simulink model "ForceMeasurement"  (R2018a)
settings: Solver=ode4  StartTime=0.0  StopTime=inf  FixedStep=0.002  RelTol=1e-3  EnableMultiTasking=on
PostLoadFcn:
  | qc_set_target_type(getConfigSet(bdroot, 'QUARC Default Target Configuration'));
undefined symbols (not defined in the file or in its folder): HIL
libraries: quarc_library x9
Description:
  | This example is a simple analog loopback test. It sends a signal to analog output
  | channel #0 and then reads analog input channel #0. Wire analog output #0 to analog
  | input #0 to see the signal on the Scope. Change the amplitude of the signal and see
  | the change occur on the Scope.
settings Model: SimulationMode=external  ExtModeTrigDuration=10000  Creator=drmadill  LastModifiedBy=dogro
settings SolverCC: PositivePriorityOrder=on
settings DataIOCC: LimitDataPoints=on  SaveFormat=Array  SignalLoggingSaveFormat=ModelDataLogs
settings OptimizationCC: ExpressionDepthLimit=2147483647  InitFltsAndDblsToZero=on  LifeSpan=inf
settings DebuggingCC: SaveWithParameterizedLinksMsg=none  UnderspecifiedInitializationDetection=Classic  MergeDetectMultiDrivingBlocksExec=none  SolverPrmCheckMsg=warning  FcnCallInpInsideContextMsg=warning  StateNameClashWarn=warning  SFUnexpectedBacktrackingDiag=warning  SFNoUnconditionalDefaultTransitionDiag=warning  SFExecutionAtInitializationDiag=none
settings HardwareCC: ProdBitPerPointer=32  ProdBitPerSizeT=32  ProdBitPerPtrDiffT=32  ProdLargestAtomicFloat=None  ProdIntDivRoundTo=Undefined  ProdEndianess=Unspecified  ProdWordSize=32  ProdHWDeviceType=32-bit Generic
settings ModelReferenceCC: PropagateSignalLabelsOutOfModel=off
settings RTWCC: SystemTargetFile=quarc_win64.tlc  TemplateMakefile=quarc_default_tmf  Description=QUARC Win64 Target
settings CodeAppCC: StateflowObjectComments=on
settings STFCustomTargetCC: TargetPreCompLibLocation=C:\PROGRA~3\QUARC\lib\2018a\win64\release  ConcurrentExecutionCompliant=on  GeneratePreprocessorConditionals=Disable all  CPPClassGenCompliant=on  SystemTargetFile=quarc_win64.tlc
settings GRTTargetCC: TargetPreCompLibLocation=C:\PROGRA~3\QUARC\lib\2018a\win64\release  TargetLangStandard=C89/C90 (ANSI)  ParMdlRefBuildCompliant=off  CompOptLevelCompliant=off  GeneratePreprocessorConditionals=Disable all  CombineOutputUpdateFcns=off  MatFileLogging=off  GRTInterface=on  UseToolchainInfoCompliant=off  ExtMode=on  ExtModeMexFile=quarc_comm
settings ConfigComp: CovMetricSettings=dw  CovHtmlReporting=on  CovSaveCumulativeToWorkspaceVar=on  CovSaveSingleToWorkspaceVar=on  CovExternalEMLEnable=off

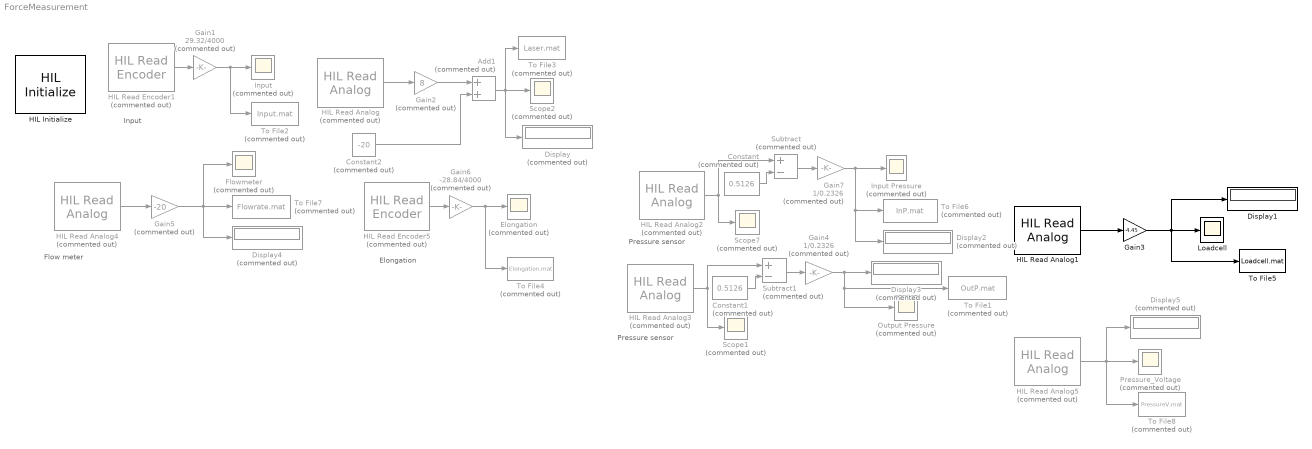
== system ForceMeasurement ==
  note: Elongation
  note: Input
  note: Pressure sensor
  note: Pressure sensor
  note: Flow meter
  Add1 : Sum  Commented=on
  Constant : Constant  Commented=on  Value=0.5126
  Constant1 : Constant  Commented=on  Value=0.5126
  Constant2 : Constant  Commented=on  Value=-20
  Display{,2..5} (5 alike) : Display  Commented=on
  Display1 : Display
  Elongation : Scope  Commented=on
  Flowmeter : Scope  Commented=on
  Gain1 : Gain  Commented=on  Gain=29.32/4000
  Gain2 : Gain  Commented=on  Gain=8
  Gain3 : Gain  Gain=-4.45
  Gain4 : Gain  Commented=on  Gain=1/0.2326
  Gain5 : Gain  Commented=on  Gain=-20
  Gain6 : Gain  Commented=on  Gain=-28.84/4000
  Gain7 : Gain  Commented=on  Gain=1/0.2326
  HIL Initialize : quarc_library/Data Acquisition/Generic/Configuration/HIL Initialize  Priority=-99  object_name=HIL-1  board_type=qpid_e  board_number=0  board_options=enc0_dir=0;enc0_filter=1;enc0_a=1;enc0_b=1;enc0_z=0;enc0_reload=0;enc1_dir=0;enc1_filter=1;enc1_a=1;enc1_b=1;enc1_z=0;enc1_reload=0;enc2_dir=0;enc2_filter=1;enc2_a=1;enc2_b=1;enc2_z=0;enc2_reload=0;enc3_dir=0;enc3_filter=1;enc3_a=1;enc3_b=1;enc3_z=0;enc3_reload=0;enc4_dir=0;enc4_filter=1;enc4_a=1;enc4_b=1;enc4_z=0;enc4_reload=0;enc5_dir=0;enc5_filter=1;enc5_a=1;enc5_b=1;enc5_z=0;enc5_reload=0;enc6_dir=0;enc6_filter=1;enc6_a=1;enc6_b=1;enc6_z=0;enc6_reload=0;enc7_dir=0;enc7_filter=1;enc7_a=1;enc7_b=1;enc7_z=0;enc7_reload=0;ext_int_polarity=0;fuse_polarity=0;convert_polarity=0;watchdog_polarity=0;ext_int_watchdog=0;fuse_watchdog=0;trig1_watchdog=0;watchdog_to_trig1=0;watchdog_to_trig2=0;counter_to_trig0=0;trigger_adcs=0;latch_on_adc=0;pwm_immediate=0  exclusive=off  active=off  hardware_clocks=[0:16]  clock_modes=[]  initial_clock_frequencies=[]  set_clock_params_at_start=off  set_clock_params_at_switch_in=off  set_clock_frequencies_at_start=off  set_clock_frequencies_at_switch_in=off  analog_input_channels=[0:7]  analog_input_configurations=[]  analog_input_maximums=10  analog_input_minimums=-10  set_analog_input_params_at_start=off  set_analog_input_params_at_switch_in=off  analog_output_channels=[0:7]  analog_output_maximums=10  analog_output_minimums=-10  initial_analog_outputs=[0]  final_analog_outputs=[0]  watchdog_analog_outputs=0  set_analog_output_params_at_start=off  set_analog_output_params_at_switch_in=off  set_analog_outputs_at_start=on  set_analog_outputs_at_switch_in=off  set_analog_outputs_at_terminate=on  set_analog_outputs_at_switch_out=off  set_analog_outputs_on_watchdog=off  digital_input_channels=[]  digital_output_channels=[]  digital_output_configuration=[]  initial_digital_outputs=[1]  final_digital_outputs=[1]  watchdog_digital_outputs=[2]  set_digital_output_params_at_start=off  set_digital_output_params_at_switch_in=off  set_digital_outputs_at_start=on  set_digital_outputs_at_switch_in=off  set_digital_outputs_at_terminate=on  set_digital_outputs_at_switch_out=off  set_digital_outputs_on_watchdog=off  encoder_channels=[0:7]  quadrature=[4]  encoder_filter_frequency=40e6/1  initial_encoder_counts=[0]  set_encoder_params_at_start=on  set_encoder_params_at_switch_in=off  set_encoder_counts_at_start=on  set_encoder_counts_at_switch_in=off  pwm_channels=[0:7]  pwm_modes=0  pwm_frequency=40e6/4096  pwm_configuration=[0]  pwm_alignment=[0]  pwm_polarity=[1]  pwm_leading_deadband=[0]  pwm_trailing_deadband=[0]  initial_pwm_outputs=[0]  final_pwm_outputs=[0]  watchdog_pwm_outputs=[0]  set_pwm_params_at_start=on  set_pwm_params_at_switch_in=off  set_pwm_outputs_at_start=on  set_pwm_outputs_at_switch_in=off  set_pwm_outputs_at_terminate=on  set_pwm_outputs_at_switch_out=off  set_pwm_outputs_on_watchdog=off  other_output_channels=[]  initial_other_outputs=[]  final_other_outputs=[]  watchdog_other_outputs=[]  set_other_outputs_at_start=off  set_other_outputs_at_switch_in=off  set_other_outputs_at_terminate=off  set_other_outputs_at_switch_out=off  set_other_outputs_on_watchdog=off
  HIL Read Analog : quarc_library/Data Acquisition/Generic/Immediate I//O/HIL Read Analog  Commented=on  object_name=HIL-1  channels=0  sample_time=qc_get_step_size  active=on  vector_output=off
  HIL Read Analog1 : quarc_library/Data Acquisition/Generic/Immediate I//O/HIL Read Analog  object_name=HIL-1  channels=[6]  sample_time=qc_get_step_size  active=on  vector_output=off
  HIL Read Analog2 : quarc_library/Data Acquisition/Generic/Immediate I//O/HIL Read Analog  Commented=on  object_name=HIL-1  channels=[0]  sample_time=qc_get_step_size  active=on  vector_output=off
  HIL Read Analog3 : quarc_library/Data Acquisition/Generic/Immediate I//O/HIL Read Analog  Commented=on  object_name=HIL-1  channels=[1]  sample_time=qc_get_step_size  active=on  vector_output=off
  HIL Read Analog4 : quarc_library/Data Acquisition/Generic/Immediate I//O/HIL Read Analog  Commented=on  object_name=HIL-1  channels=[2]  sample_time=qc_get_step_size  active=on  vector_output=off
  HIL Read Analog5 : quarc_library/Data Acquisition/Generic/Immediate I//O/HIL Read Analog  Commented=on  object_name=HIL-1  channels=[1]  sample_time=qc_get_step_size  active=on  vector_output=off
  HIL Read Encoder1 : quarc_library/Data Acquisition/Generic/Immediate I//O/HIL Read Encoder  Commented=on  object_name=HIL-1  channels=[1]  sample_time=qc_get_step_size  active=on  vector_output=off  data_type_mode=Inherit via back propagation  data_type=double
  HIL Read Encoder5 : quarc_library/Data Acquisition/Generic/Immediate I//O/HIL Read Encoder  Commented=on  object_name=HIL-1  channels=[1]  sample_time=qc_get_step_size  active=on  vector_output=off  data_type_mode=Inherit via back propagation  data_type=double
  Input : Scope  Commented=on
  Input Pressure : Scope  Commented=on
  Loadcell : Scope
  Output Pressure : Scope  Commented=on
  Pressure_Voltage : Scope  Commented=on
  Scope1 : Scope  Commented=on
  Scope2 : Scope  Commented=on
  Scope7 : Scope  Commented=on
  Subtract : Sum  Commented=on  Inputs=+-
  Subtract1 : Sum  Commented=on  Inputs=+-
  To File1 : ToFile  Commented=on  Filename=OutP.mat  MatrixName=OutPressure
  To File2 : ToFile  Commented=on  Filename=Input.mat  MatrixName=Input
  To File3 : ToFile  Commented=on  Filename=Laser.mat  MatrixName=Laser
  To File4 : ToFile  Commented=on  Filename=Elongation.mat  MatrixName=Elongation
  To File5 : ToFile  Filename=Loadcell.mat  MatrixName=Loadcell
  To File6 : ToFile  Commented=on  Filename=InP.mat  MatrixName=InPressure
  To File7 : ToFile  Commented=on  Filename=Flowrate.mat  MatrixName=Flowrate
  To File8 : ToFile  Commented=on  Filename=PressureV.mat  MatrixName=PressureV
  wires:
  HIL Read Encoder5/1 -> Gain6/1
  Gain6/1 -> Elongation/1, To File4/1
  Gain1/1 -> Input/1, To File2/1
  HIL Read Encoder1/1 -> Gain1/1
  Constant2/1 -> Add1/2
  HIL Read Analog/1 -> Gain2/1
  Gain2/1 -> Add1/1
  Add1/1 -> To File3/1, Display/1, Scope2/1
  HIL Read Analog1/1 -> Gain3/1
  Gain3/1 -> To File5/1, Loadcell/1, Display1/1
  Constant/1 -> Subtract/2
  HIL Read Analog2/1 -> Subtract/1, Scope7/1
  Subtract/1 -> Gain7/1
  Gain7/1 -> Display2/1, To File6/1, Input Pressure/1
  Gain4/1 -> Output Pressure/1, To File1/1, Display3/1
  HIL Read Analog3/1 -> Subtract1/1, Scope1/1
  Constant1/1 -> Subtract1/2
  Subtract1/1 -> Gain4/1
  Gain5/1 -> Flowmeter/1, Display4/1, To File7/1
  HIL Read Analog4/1 -> Gain5/1
  HIL Read Analog5/1 -> Display5/1, To File8/1, Pressure_Voltage/1
